simulink model "drivePMSM"  (R2024b)
settings: Solver=VariableStepAuto  StartTime=0.0  StopTime=0.05  MaxStep=1e-3  RelTol=1e-3
undefined symbols (not defined in the file or in its folder): inverter, mot
settings Model: Creator=giulio  LastModifiedBy=giulio

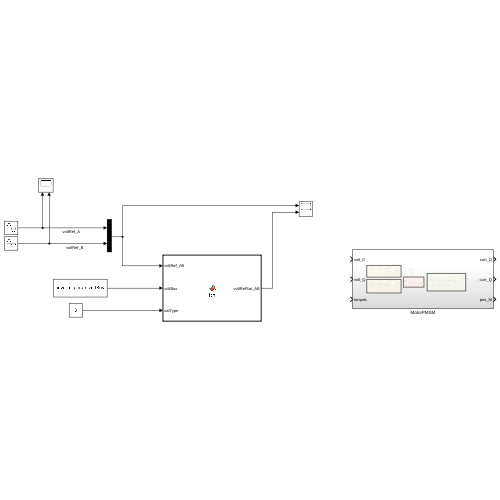
[thumbnail: Simulink's stored preview of the top-level diagram]
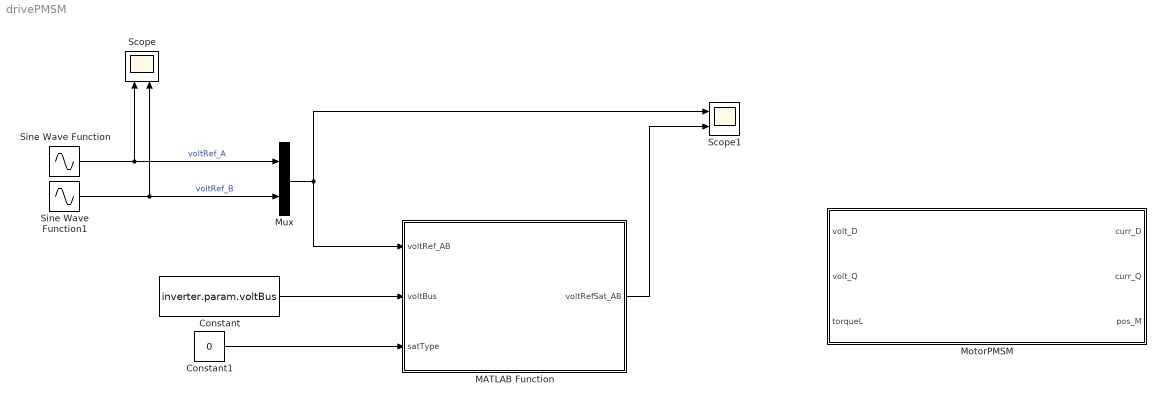
== system drivePMSM ==
  Constant : Constant  Value=inverter.param.voltBus
  Constant1 : Constant  Value=0
  MATLAB Function : MATLAB Function  TreatAsAtomicUnit=on
  MotorPMSM : Subsystem
  Mux : Mux  Inputs=2
  Scope : Scope  NumInputPorts=2
  Scope1 : Scope  NumInputPorts=2
  Sine Wave Function : Sin  Amplitude=24  Frequency=50*2*pi  SampleTime=0
  Sine Wave Function1 : Sin  Amplitude=24  Frequency=50*2*pi  Phase=pi/2  SampleTime=0
  wires:
  Constant/1 -> MATLAB Function/2(voltBus)
  Constant1/1 -> MATLAB Function/3(satType)
  Mux/1 -> MATLAB Function/1(voltRef_AB), Scope1/1
  Sine Wave Function/1 -> Mux/1, Scope/1  "voltRef_A"
  Sine Wave Function1/1 -> Mux/2, Scope/2  "voltRef_B"
  MATLAB Function/1(voltRefSat_AB) -> Scope1/2

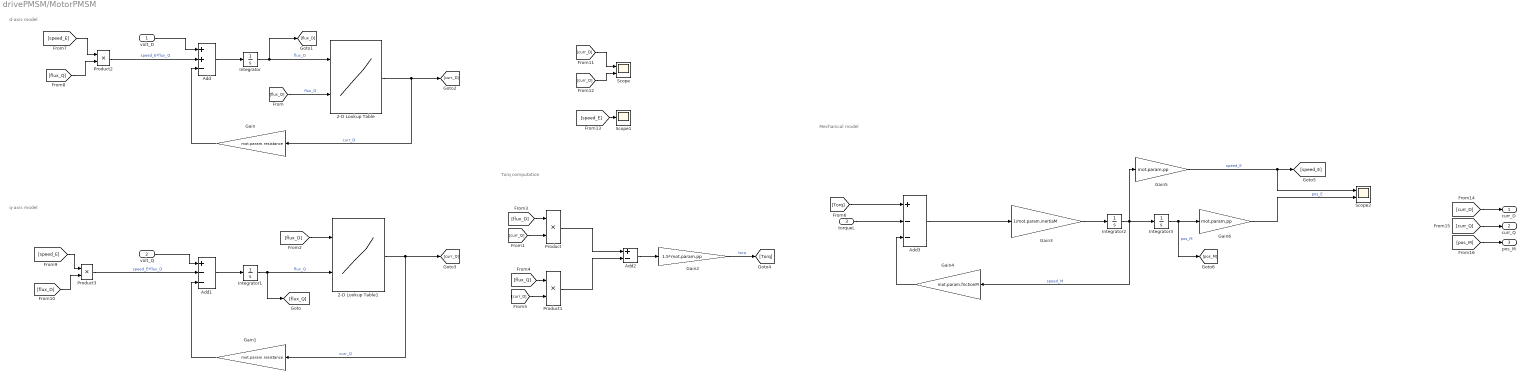
== system drivePMSM/MotorPMSM ==
  note: Mechanical model
  note: Torq computation
  note: d-axis model
  note: q-axis model
  volt_D : Inport
  volt_Q : Inport  Port=2
  torqueL : Inport  Port=3
  2-D Lookup Table : Lookup_n-D  BreakpointsForDimension1=mot.maps.fluxVec_D  BreakpointsForDimension2=mot.maps.fluxVec_Q  Table=mot.maps.currMap_D'  InternalRulePriority=Speed  RndMeth=Simplest
      settings: InputPortMap=u0,u1
  2-D Lookup Table1 : Lookup_n-D  BreakpointsForDimension1=mot.maps.fluxVec_D  BreakpointsForDimension2=mot.maps.fluxVec_Q  Table=mot.maps.currMap_Q'  InternalRulePriority=Speed  RndMeth=Simplest
      settings: InputPortMap=u0,u1
  Add : Sum  Inputs=++-
  Add1 : Sum  Inputs=+--
  Add2 : Sum  Inputs=+-
  Add3 : Sum  Inputs=+--
  Gain : Gain  Gain=mot.param.resistance
  Gain1 : Gain  Gain=mot.param.resistance
  Gain2 : Gain  Gain=1.5*mot.param.pp
  Gain3 : Gain  Gain=1/mot.param.inertiaM
  Gain4 : Gain  Gain=mot.param.frictionM
  Gain5 : Gain  Gain=mot.param.pp
  Gain6 : Gain  Gain=mot.param.pp
  Integrator : Integrator  InitialCondition=mot.param.fluxPM
  Integrator1 : Integrator
  Integrator2 : Integrator
  Integrator3 : Integrator
  Product{,1..3} (4 alike) : Product
  Scope : Scope  NumInputPorts=2
  Scope1 : Scope
  Scope2 : Scope  NumInputPorts=2
  curr_D : Outport
  curr_Q : Outport  Port=2
  pos_M : Outport  Port=3
  wires:
  [flux_Q] -> Product1/1
  [speed_E] -> Scope1/1
  Integrator3/1 -> [pos_M], Gain6/1  "pos_M"
  Add2/1 -> Gain2/1
  Gain5/1 -> Scope2/1, [speed_E]  "speed_E"
  Product/1 -> Add2/1
  Integrator/1 -> [flux_D], 2-D Lookup Table/1  "flux_D"
  Product3/1 -> Add1/2  "speed_E*flux_D"
  Gain4/1 -> Add3/3
  [flux_D] -> Product3/2
  volt_D/1 -> Add/1
  Add/1 -> Integrator/1
  [flux_D] -> 2-D Lookup Table1/1
  Gain/1 -> Add/3
  Integrator2/1 -> Gain5/1, Gain4/1, Integrator3/1  "speed_M"
  Add1/1 -> Integrator1/1
  Gain1/1 -> Add1/3
  [flux_D] -> Product/1
  Add3/1 -> Gain3/1
  [curr_Q] -> Product/2
  Gain6/1 -> Scope2/2  "pos_E"
  Integrator1/1 -> [flux_Q], 2-D Lookup Table1/2  "flux_Q"
  Gain2/1 -> [Torq]  "torq"
  Gain3/1 -> Integrator2/1
  [flux_Q] -> Product2/2
  [curr_D] -> Scope/1
  [curr_Q] -> Scope/2
  torqueL/1 -> Add3/2
  [curr_D] -> Product1/2
  [flux_Q] -> 2-D Lookup Table/2  "flux_Q"
  2-D Lookup Table1/1 -> [curr_Q], Gain1/1  "curr_Q"
  Product2/1 -> Add/2  "speed_E*flux_Q"
  Product1/1 -> Add2/2
  volt_Q/1 -> Add1/1
  2-D Lookup Table/1 -> [curr_D], Gain/1  "curr_D"
  [Torq] -> Add3/1
  [speed_E] -> Product3/1
  [speed_E] -> Product2/1
  [pos_M] -> pos_M/1
  [curr_Q] -> curr_Q/1
  [curr_D] -> curr_D/1

== matlab function drivePMSM/MATLAB Function ==
  data: voltRef_AB input; voltRefSat_AB output; voltBus input; satType input; inverter parameter
function voltRefSat_AB = fcn(voltRef_AB,voltBus,satType,inverter)
%satType = 0 -> circular saturation 
%satType = 1 -> hexagonal saturation 

Tpwm = inverter.param.timePWM;

%% Circular saturation 
voltRefMag_AB = sqrt(voltRef_AB(1)^2+voltRef_AB(2)^2);
voltBus_sqrt3 = voltBus / sqrt(3);

if ((satType == 0) && (voltRefMag_AB > voltBus_sqrt3))
    %Circular saturation 
    k_sat = voltBus_sqrt3 / voltRefMag_AB;
    voltRefSat_AB = voltRef_AB * k_sat;
else
    voltRefSat_AB = voltRef_AB;
end

%% Sector identification
if (voltRefSat_AB(2) >= 0) %1,2 o 3 sector
    if(voltRefSat_AB(1) >= 0) %1 o 2 sector
        if(voltRefSat_AB(1)*sqrt(3) > voltRefSat_AB(2)) % 1 sector
            m = 1;
        else 
            m = 2;
        end
    else 
        if(voltRefSat_AB(1)*(-sqrt(3)) <= voltRefSat_AB(2))
            m = 2;
        else 
            m = 3;
        end

    end
else % 4,5,6 sector 
    if(voltRefSat_AB(1) < 0) %4 o 5 sector
        if(voltRefSat_AB(1)*-sqrt(3) > -voltRefSat_AB(2))
            m = 4;
        else 
            m = 5;
        end
    else 
        if(voltRefSat_AB(1)*(sqrt(3)) <= -voltRefSat_AB(2))
            m = 5;
        else 
            m = 6;
        end

    end

end

%% Time vector application

k_T = sqrt(3) * Tpwm/voltBus;


T1 =  k_T * (voltRefSat_AB(1) * sin(m*pi/3) - voltRefSat_AB(2) * cos(m * pi/3));
T2 =  k_T * (-voltRefSat_AB(1) * sin((m-1)*pi/3) + voltRefSat_AB(2) * cos((m-1) * pi/3));

% get null vector time 
T0 = Tpwm - T1 - T2;


%% Check hexagonal saturation

if(T0 < 0)
    % hexagonal saturation 
    k_sat = Tpwm/(T1+T2);
    T1 = T1 * k_sat;
    T2 = T2 * k_sat;
    %saturate voltages 
    voltRefSat_AB = voltRefSat_AB*k_sat;
end
